simulink model "traffic_light_model_1"  (R2024b)
settings: Solver=ode4  StartTime=0.0  StopTime=300  FixedStep=0.1  RelTol=1e-3
undefined symbols (not defined in the file or in its folder): DiscIntNeverNeededParam
libraries: simulink x1
settings Model: Creator=curicae  LastModifiedBy=curicae

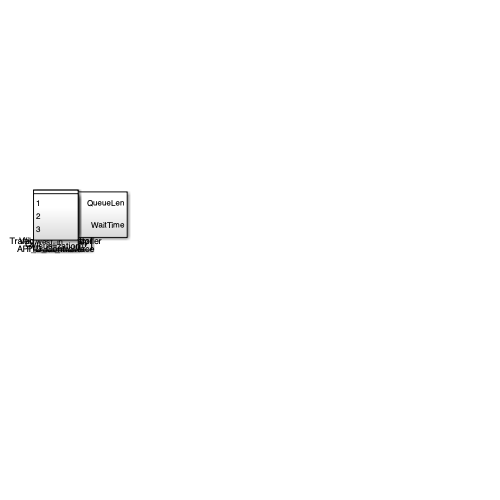
[thumbnail: Simulink's stored preview of the top-level diagram]
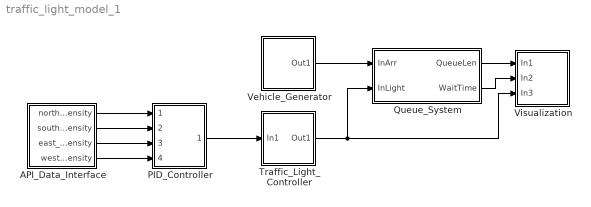
== system traffic_light_model_1 ==
  API_Data_Interface : Subsystem
  PID_Controller : Subsystem
  Queue_System : Subsystem
  Traffic_Light_Controller : Subsystem
  Vehicle_Generator : Subsystem
  Visualization : Subsystem
  wires:
  Queue_System/1(QueueLen) -> Visualization/1(In1)
  Queue_System/2(WaitTime) -> Visualization/2(In2)
  Traffic_Light_Controller/1(Out1) -> Queue_System/2(InLight), Visualization/3(In3)
  Vehicle_Generator/1(Out1) -> Queue_System/1(InArr)
  API_Data_Interface/4(west_density) -> PID_Controller/4(west_in)
  API_Data_Interface/3(east_density) -> PID_Controller/3(east_in)
  API_Data_Interface/2(south_density) -> PID_Controller/2(south_in)
  PID_Controller/1(Out1) -> Traffic_Light_Controller/1(In1)
  API_Data_Interface/1(north_density) -> PID_Controller/1(north_in)

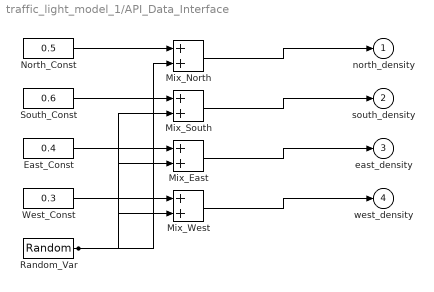
== system traffic_light_model_1/API_Data_Interface ==
  East_Const : Constant  Value=0.4
  Mix_East : Sum
  Mix_North : Sum
  Mix_South : Sum
  Mix_West : Sum
  North_Const : Constant  Value=0.5
  Random_Var : UniformRandomNumber  Minimum=-0.1  Maximum=0.1  SampleTime=0.1
  South_Const : Constant  Value=0.6
  West_Const : Constant  Value=0.3
  north_density : Outport
  south_density : Outport  Port=2
  east_density : Outport  Port=3
  west_density : Outport  Port=4
  wires:
  North_Const/1 -> Mix_North/1
  South_Const/1 -> Mix_South/1
  East_Const/1 -> Mix_East/1
  West_Const/1 -> Mix_West/1
  Random_Var/1 -> Mix_North/2, Mix_South/2, Mix_East/2, Mix_West/2
  Mix_North/1 -> north_density/1
  Mix_South/1 -> south_density/1
  Mix_East/1 -> east_density/1
  Mix_West/1 -> west_density/1

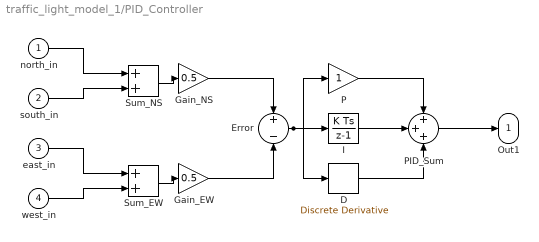
== system traffic_light_model_1/PID_Controller ==
  north_in : Inport
  south_in : Inport  Port=2
  east_in : Inport  Port=3
  west_in : Inport  Port=4
  D : simulink/Discrete/Discrete Derivative  gainval=1.0  ICPrevScaledInput=0.0  OutMin=[]  OutMax=[]  OutDataType=fixdt(1, 16)  OutScaling=2^-10  DoSatur=off
  Error : Sum  Inputs=+-
  Gain_EW : Gain  Gain=0.5
  Gain_NS : Gain  Gain=0.5
  I : DiscreteIntegrator  SampleTime=-1  ICPrevOutput=DiscIntNeverNeededParam  ICPrevScaledInput=DiscIntNeverNeededParam
  P : Gain
  PID_Sum : Sum  Inputs=+++
  Sum_EW : Sum
  Sum_NS : Sum
  Out1 : Outport
  wires:
  north_in/1 -> Sum_NS/1
  south_in/1 -> Sum_NS/2
  Sum_NS/1 -> Gain_NS/1
  east_in/1 -> Sum_EW/1
  west_in/1 -> Sum_EW/2
  Sum_EW/1 -> Gain_EW/1
  Gain_NS/1 -> Error/1
  Gain_EW/1 -> Error/2
  Error/1 -> P/1, I/1, D/1
  P/1 -> PID_Sum/1
  I/1 -> PID_Sum/2
  D/1 -> PID_Sum/3
  PID_Sum/1 -> Out1/1

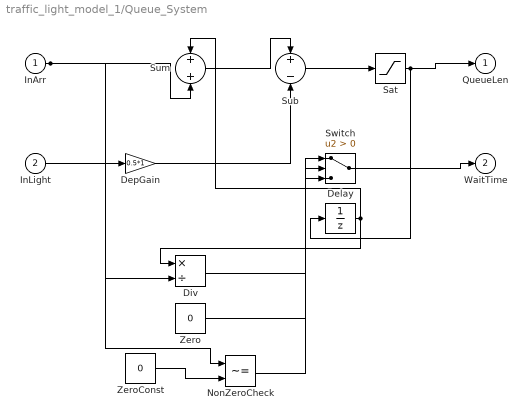
== system traffic_light_model_1/Queue_System ==
  InArr : Inport
  InLight : Inport  Port=2
  Delay : UnitDelay  SampleTime=-1  HasFrameUpgradeWarning=on
  DepGain : Gain  Gain=0.5*1
  Div : Product  Inputs=*/
  NonZeroCheck : RelationalOperator  Operator=~=  OutDataTypeStr=boolean  RndMeth=Simplest  InputSameDT=off
  Sat : Saturate  UpperLimit=100  LowerLimit=0
  Sub : Sum  Inputs=+-
  Sum : Sum
  Switch : Switch  Criteria=u2 > Threshold  SaturateOnIntegerOverflow=off  InputSameDT=off
  Zero : Constant  Value=0
  ZeroConst : Constant  Value=0
  QueueLen : Outport
  WaitTime : Outport  Port=2
  wires:
  InLight/1 -> DepGain/1
  Delay/1 -> Sum/1, Div/1
  InArr/1 -> Sum/2, Div/2, NonZeroCheck/1
  Sum/1 -> Sub/1
  DepGain/1 -> Sub/2
  Sub/1 -> Sat/1
  Sat/1 -> Delay/1, QueueLen/1
  Div/1 -> Switch/1
  ZeroConst/1 -> NonZeroCheck/2
  NonZeroCheck/1 -> Switch/2
  Zero/1 -> Switch/3
  Switch/1 -> WaitTime/1

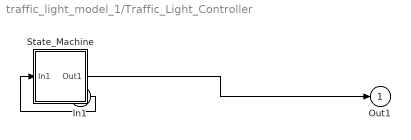
== system traffic_light_model_1/Traffic_Light_Controller ==
  In1 : Inport
  State_Machine : Subsystem
  Out1 : Outport
  wires:
  In1/1 -> State_Machine/1(In1)
  State_Machine/1(Out1) -> Out1/1

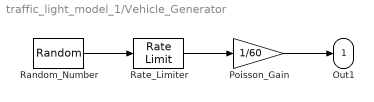
== system traffic_light_model_1/Vehicle_Generator ==
  Poisson_Gain : Gain  Gain=1/60
  Random_Number : UniformRandomNumber  Minimum=0  SampleTime=0.1
  Rate_Limiter : RateLimiter
  Out1 : Outport
  wires:
  Random_Number/1 -> Rate_Limiter/1
  Rate_Limiter/1 -> Poisson_Gain/1
  Poisson_Gain/1 -> Out1/1

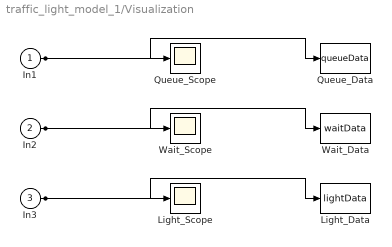
== system traffic_light_model_1/Visualization ==
  In1 : Inport
  In2 : Inport  Port=2
  In3 : Inport  Port=3
  Light_Data : ToWorkspace  VariableName=lightData  SaveFormat=Timeseries  SampleTime=-1
  Light_Scope : Scope
  Queue_Data : ToWorkspace  VariableName=queueData  SaveFormat=Timeseries  SampleTime=-1
  Queue_Scope : Scope
  Wait_Data : ToWorkspace  VariableName=waitData  SaveFormat=Timeseries  SampleTime=-1
  Wait_Scope : Scope
  wires:
  In1/1 -> Queue_Scope/1, Queue_Data/1
  In2/1 -> Wait_Scope/1, Wait_Data/1
  In3/1 -> Light_Scope/1, Light_Data/1

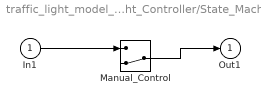
== system traffic_light_model_1/Traffic_Light_Controller/State_Machine ==
  In1 : Inport
  Manual_Control : ManualSwitch  CurrentSetting=0
  Out1 : Outport
  wires:
  In1/1 -> Manual_Control/1
  Manual_Control/1 -> Out1/1
